simulink model "Hybrid_vehicle"  (R2020a)
settings: Solver=VariableStepAuto  StartTime=0.0  StopTime=1800  MaxStep=0.05  RelTol=1e-8
values from neighbouring files (symbols this model uses):
  Bdy_facTireFric_C = 0.018    [Model_parameters.mat]
  Bdy_lenRadiusWheel_C = 0.32    [Model_parameters.mat]
  Bdy_mEquivalentJ_C = 60    [Model_parameters.mat]
  Bdy_mVeh_C = 1400    [Model_parameters.mat]
  Bdy_vsqr2frc_C = 0.429    [Model_parameters.mat]
  Drv_facSlopeWLTC_CUR = [0 500 1000 1500 2000 2500 3000 3500 4000 4500 5000 5500 ... (98 elements, 49x2)]    [Model_parameters.mat]
  Drv_kmh2gradtqDriver_C = 200    [Model_parameters.mat]
  Drv_kmh2tqDriver_C = 500    [Model_parameters.mat]
  Drv_kmhDesWLTC_CUR = [1 2 3 4 5 6 7 8 9 10 11 12 ... (3600 elements, 1800x2)]    [Model_parameters.mat]
  Edr_pwr_LossMap_AXIS = [-150000 -100000 -60000 -35000 -23000 -7000 -2000 -1000 -200 0 200 1000 ... (19 elements, 1x19)]    [Model_parameters.mat]
  Edr_pwrInverterLosses_MAP = [19500 13000 6600 3500 2990 1470 600 450 160 50 160 450 ... (76 elements, 19x4)]    [Model_parameters.mat]
  Edr_pwrMachineLosses_MAP = [330 270 210 150 120 90 60 30 10 0 20 40 ... (209 elements, 19x11)]    [Model_parameters.mat]
  Edr_rpm_InvLossMap_AXIS = [0 2000 5000 12000]    [Model_parameters.mat]
  Edr_rpm_MachLossMap_AXIS = [0 100 200 400 1000 2000 4000 6000 8000 10000 12000]    [Model_parameters.mat]
  Edr_rpm_MaxMinTq_AXIS = [0 100 200 400 1000 2000 4000 5000 6000 7000 8000 10000 ... (13 elements, 13x1)]    [Model_parameters.mat]
  Edr_tq_MachLossMap_AXIS = [-220 -180 -140 -100 -80 -60 -40 -20 -10 0 10 20 ... (19 elements, 1x19)]    [Model_parameters.mat]
  Edr_tqEffMax_CUR = [220 220 220 220 220 220 220 180 150 125 106 81 ... (13 elements, 13x1)]    [Model_parameters.mat]
  GbxFr_tqClutchMax_C = 500    [Model_parameters.mat]
  GbxRe_facGbxReRatio_C = 10    [Model_parameters.mat]
  Ice_derfacLoadDecrease_MAP = [-5 -200 -225 -250 -275 -300 -325 -350 -375 -400 -10 -400 ... (120 elements, 10x12)]    [Model_parameters.mat]
  Ice_derfacLoadIncrease_MAP = [500 30 30 30 30 30 0 0 0 0 500 50 ... (120 elements, 10x12)]    [Model_parameters.mat]
  Ice_facEtaCocMax_MAP = [1 1 0.98 0.955 0.93 1 1 0.986 0.965 0.94 1 1 ... (35 elements, 5x7)]    [Model_parameters.mat]
  Ice_facFuelEnRich_MAP = [1 1 1 1 1 1 1 1 1 1.02 1 1 ... (35 elements, 5x7)]    [Model_parameters.mat]
  Ice_Load2TqOptIgnLamOne_MAP = [0 35 70 105 140 0 38 76 114 152 0 40 ... (35 elements, 5x7)]    [Model_parameters.mat]
  Ice_relLoad_AXIS = [0 40 80 120 160]    [Model_parameters.mat]
  Ice_relLoad_LoadDyn_AXIS = [0 80 90 100 110 120 130 140 150 160]    [Model_parameters.mat]
  Ice_relLoad_Max_CUR = [50 130 137 143 148 153 159 160 160 157 130 90]    [Model_parameters.mat]
  Ice_rpm_AXIS = [0 1000 2000 3000 4000 5000 6000]    [Model_parameters.mat]
  Ice_rpm_LoadDyn_AXIS = [500 1000 1100 1200 1300 1400 1600 2400 3000 4000 5000 6000]    [Model_parameters.mat]
  Ice_tq_AXIS = [0 40 80 120 160]    [Model_parameters.mat]
  Ice_tqLossesIce_MAP = [15 13 11 11 11 15 13 11 11 11 16 14 ... (35 elements, 5x7)]    [Model_parameters.mat]
  Ice_TqOptIgnLamOne2Load_MAP = [0 45.7 91.4 137.14 182.85 0 42.1 84.2 126.3 168.4 0 40 ... (35 elements, 5x7)]    [Model_parameters.mat]
  Pnt_capBat_C = 54000    [Model_parameters.mat]
  Pnt_facSocInit_C = 0.6    [Model_parameters.mat]
  Pnt_resBatInner_C = 0.2    [Model_parameters.mat]
libraries: simulink x2
(part 2 of 2)

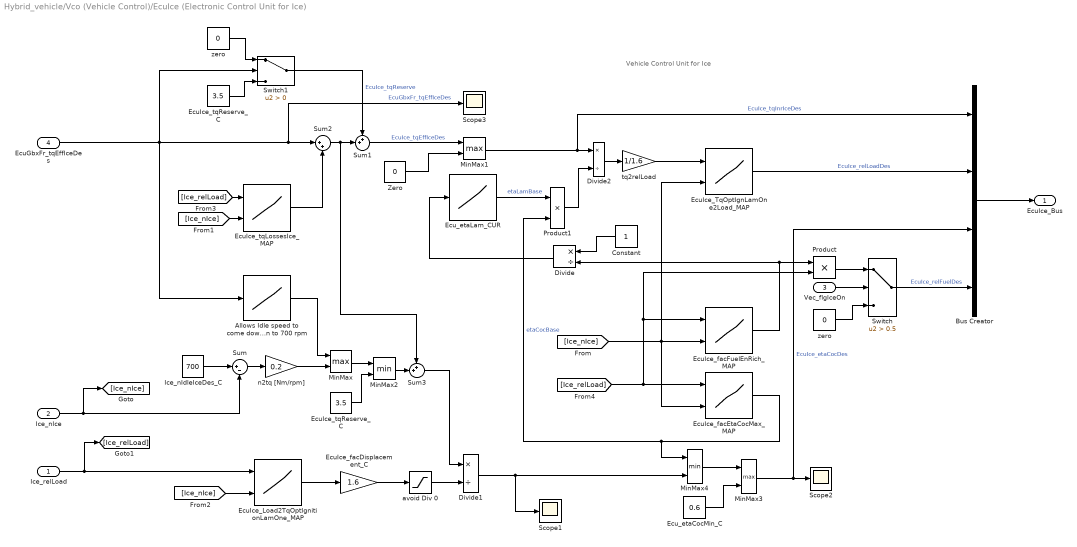
== system Hybrid_vehicle/Vco (Vehicle Control)/EcuIce (Electronic Control Unit for Ice) ==
  note: Vehicle Control Unit for Ice
  Ice_relLoad : Inport
  Ice_nIce : Inport  Port=2
  Vec_flgIceOn : Inport  Port=3
  EcuGbxFr_tqEffIceDes : Inport  Port=4
  " zero " : Constant  Value=0
  Allows Idle speed to come down to 700 rpm : Lookup_n-D  NumberOfTableDimensions=1  BreakpointsForDimension1="[-1 0  1  2]"  Table=[-1 -1 0 0 ]  InternalRulePriority=Speed  RndMeth=Simplest  InputSameDT=on
  Bus Creator : BusCreator  Inputs=4
  Constant : Constant
  Divide : Product  Inputs=*/
  Divide1 : Product  Inputs=*/
  Divide2 : Product  Inputs=*/
  EcuIce_Load2TqOptIgnitionLamOne_MAP : Lookup_n-D  BreakpointsForDimension1=Ice_relLoad_AXIS  BreakpointsForDimension2=Ice_rpm_AXIS  Table=Ice_Load2TqOptIgnLamOne_MAP  ExtrapMethod=Clip  InternalRulePriority=Speed  RndMeth=Simplest  InputSameDT=on
  EcuIce_TqOptIgnLamOne2Load_MAP : Lookup_n-D  BreakpointsForDimension1=Ice_tq_AXIS  BreakpointsForDimension2=Ice_rpm_AXIS  Table=Ice_TqOptIgnLamOne2Load_MAP  ExtrapMethod=Clip  InternalRulePriority=Speed  RndMeth=Simplest  InputSameDT=on
  EcuIce_facDisplacement_C : Gain  Gain=1.6
  EcuIce_facEtaCocMax_MAP : Lookup_n-D  BreakpointsForDimension1=Ice_relLoad_AXIS  BreakpointsForDimension2=Ice_rpm_AXIS  Table=Ice_facEtaCocMax_MAP  ExtrapMethod=Clip  InternalRulePriority=Speed  RndMeth=Simplest  InputSameDT=on
  EcuIce_facFuelEnRich_MAP : Lookup_n-D  BreakpointsForDimension1=Ice_relLoad_AXIS  BreakpointsForDimension2=Ice_rpm_AXIS  Table=Ice_facFuelEnRich_MAP  ExtrapMethod=Clip  InternalRulePriority=Speed  RndMeth=Simplest  InputSameDT=on
  EcuIce_tqLossesIce_MAP : Lookup_n-D  BreakpointsForDimension1=Ice_relLoad_AXIS  BreakpointsForDimension2=Ice_rpm_AXIS  Table=Ice_tqLossesIce_MAP  ExtrapMethod=Clip  InternalRulePriority=Speed  RndMeth=Simplest  InputSameDT=on
  EcuIce_tqReserve_C : Constant  Value=3.5
  "EcuIce_tqReserve_C " : Constant  Value=3.5
  Ecu_etaCocMin_C : Constant  Value=0.6
  Ecu_etaLam_CUR : Lookup_n-D  NumberOfTableDimensions=1  BreakpointsForDimension1="[0.5    0.6     0.7   0.8   0.85   0.9   1.0   1.1    1.2    1.3    1.4    1.5    1.6    1.7    1.8    1.9    2.0]"  Table="[0       0.5       1     1.1  1.12  1.06   1.0  0.93  0.85   0.78   0.72    0.66    0.625   0.588  0.3  0.2  0]"  ExtrapMethod=Clip  InternalRulePriority=Speed  RndMeth=Simplest  InputSameDT=on
  Ice_nIdleIceDes_C : Constant  Value=700
  MinMax : MinMax  Function=max  Inputs=2
  MinMax1 : MinMax  Function=max  Inputs=2
  MinMax2 : MinMax  Inputs=2
  MinMax3 : MinMax  Function=max  Inputs=2
  MinMax4 : MinMax  Inputs=2
  Product : Product
  Product1 : Product
  Scope1 : Scope
  Scope2 : Scope
  Scope3 : Scope
  Sum : Sum  Inputs=|+-
  Sum1 : Sum  Inputs=++|
  Sum2 : Sum  Inputs=|++
  Sum3 : Sum  Inputs=++|
  Switch : Switch  Criteria=u2 > Threshold  Threshold=0.5
  Switch1 : Switch  Criteria=u2 > Threshold
  "Zero " : Constant  Value=0
  avoid Div 0 : Saturate  UpperLimit=inf  LowerLimit=0.01
  n2tq [Nm/rpm] : Gain  Gain=0.2
  tq2relLoad : Gain  Gain=1/1.6
  "zero " : Constant  Value=0
  EcuIce_Bus : Outport  VectorParamsAs1DForOutWhenUnconnected=off
  wires:
  Bus Creator/1 -> EcuIce_Bus/1
  EcuGbxFr_tqEffIceDes/1 -> Switch1/2, Scope3/1, Sum2/1, Allows Idle speed to come down to 700 rpm/1  "EcuGbxFr_tqEffIceDes"
  Ice_nIdleIceDes_C/1 -> Sum/1
  Sum1/1 -> MinMax1/1  "EcuIce_tqEffIceDes"
  Sum3/1 -> Divide1/1
  Sum/1 -> n2tq [Nm/rpm]/1
  n2tq [Nm/rpm]/1 -> MinMax/2
  Ice_nIce/1 -> [Ice_nIce], Sum/2
  Ice_relLoad/1 -> EcuIce_Load2TqOptIgnitionLamOne_MAP/1, [Ice_relLoad]
  EcuIce_TqOptIgnLamOne2Load_MAP/1 -> Bus Creator/2  "EcuIce_relLoadDes"
  EcuIce_tqLossesIce_MAP/1 -> Sum2/2
  MinMax1/1 -> Bus Creator/1, Divide2/1  "EcuIce_tqInrIceDes"
  "Zero "/1 -> MinMax1/2
  Allows Idle speed to come down to 700 rpm/1 -> MinMax/1
  Vec_flgIceOn/1 -> Switch/2
  EcuIce_facDisplacement_C/1 -> avoid Div 0/1
  EcuIce_Load2TqOptIgnitionLamOne_MAP/1 -> EcuIce_facDisplacement_C/1
  avoid Div 0/1 -> Divide1/2
  "zero "/1 -> Switch1/1
  EcuIce_tqReserve_C/1 -> Switch1/3
  Switch1/1 -> Sum1/1  "EcuIce_tqReserve"
  Sum2/1 -> Sum3/1, Sum1/2
  Divide1/1 -> Scope1/1, MinMax4/2
  MinMax4/1 -> MinMax3/1
  Ecu_etaCocMin_C/1 -> MinMax3/2
  MinMax3/1 -> Scope2/1, Bus Creator/3  "EcuIce_etaCocDes"
  tq2relLoad/1 -> EcuIce_TqOptIgnLamOne2Load_MAP/1
  [Ice_nIce] -> EcuIce_TqOptIgnLamOne2Load_MAP/2, EcuIce_facEtaCocMax_MAP/2, EcuIce_facFuelEnRich_MAP/2
  [Ice_nIce] -> EcuIce_tqLossesIce_MAP/2
  [Ice_nIce] -> EcuIce_Load2TqOptIgnitionLamOne_MAP/2
  [Ice_relLoad] -> EcuIce_tqLossesIce_MAP/1
  MinMax/1 -> MinMax2/1
  MinMax2/1 -> Sum3/2
  "EcuIce_tqReserve_C "/1 -> MinMax2/2
  Switch/1 -> Bus Creator/4  "EcuIce_relFuelDes"
  EcuIce_facEtaCocMax_MAP/1 -> Product1/2, MinMax4/1  "etaCocBase"
  [Ice_relLoad] -> Product/2, EcuIce_facFuelEnRich_MAP/1, EcuIce_facEtaCocMax_MAP/1
  Divide2/1 -> tq2relLoad/1
  Constant/1 -> Divide/1
  Product1/1 -> Divide2/2
  Ecu_etaLam_CUR/1 -> Product1/1  "etaLamBase"
  Divide/1 -> Ecu_etaLam_CUR/1
  EcuIce_facFuelEnRich_MAP/1 -> Product/1, Divide/2
  Product/1 -> Switch/1
  " zero "/1 -> Switch/3

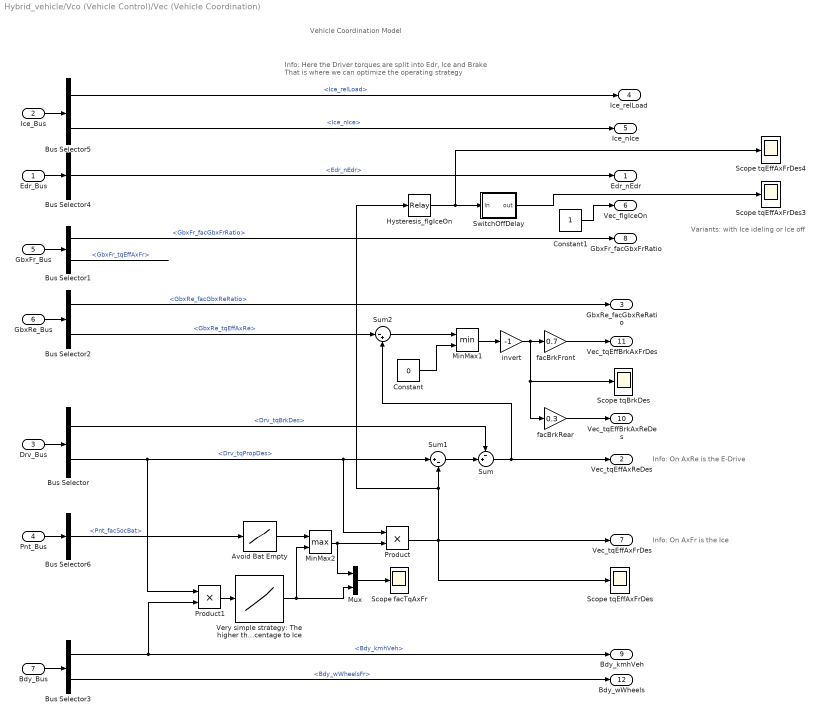
== system Hybrid_vehicle/Vco (Vehicle Control)/Vec (Vehicle Coordination) ==
  note: Vehicle Coordination Model
  note: Info: Here the Driver torques are split into Edr, Ice and Brake
      | That is where we can optimize the operating strategy
  note: Info: On AxRe is the E-Drive
  note: Info: On AxFr is the Ice
  note: Variants: with Ice ideling or Ice off
  Edr_Bus : Inport
  Ice_Bus : Inport  Port=2
  Drv_Bus : Inport  Port=3
  Pnt_Bus : Inport  Port=4
  GbxFr_Bus : Inport  Port=5
  GbxRe_Bus : Inport  Port=6
  Bdy_Bus : Inport  Port=7
  Avoid Bat Empty : Lookup_n-D  NumberOfTableDimensions=1  BreakpointsForDimension1="[0 0.1 0.2  1]"  Table="[1.1 0.8  0 0]"  InternalRulePriority=Speed  RndMeth=Simplest  InputSameDT=on
  Bus Selector : BusSelector  OutputSignals=Drv_tqBrkDes,Drv_tqPropDes
  Bus Selector1 : BusSelector  OutputSignals=GbxFr_facGbxFrRatio,GbxFr_tqEffAxFr
  Bus Selector2 : BusSelector  OutputSignals=GbxRe_facGbxReRatio,GbxRe_tqEffAxRe
  Bus Selector3 : BusSelector  OutputSignals=Bdy_kmhVeh,Bdy_wWheelsFr
  Bus Selector4 : BusSelector  OutputSignals=Edr_nEdr
  Bus Selector5 : BusSelector  OutputSignals=Ice_relLoad,Ice_nIce
  Bus Selector6 : BusSelector  OutputSignals=Pnt_facSocBat
  Constant : Constant  Value=0
  Constant1 : Constant
  Hysteresis_flgIceOn : Relay  OnSwitchValue=50  OffSwitchValue=2
  MinMax1 : MinMax  Inputs=2  ZeroCross=off
  MinMax2 : MinMax  Function=max  Inputs=2  ZeroCross=off
  Mux : Mux  Inputs=2
  Product : Product
  Product1 : Product
  Scope facTqAxFr : Scope
  Scope tqBrkDes : Scope
  Scope tqEffAxFrDes : Scope
  Scope tqEffAxFrDes3 : Scope
  Scope tqEffAxFrDes4 : Scope
  Sum : Sum  Inputs=-+|
  Sum1 : Sum  Inputs=|+-
  Sum2 : Sum  Inputs=|-+
  SwitchOffDelay : Subsystem
  "Very simple strategy: The higher the power, the more percentage to Ice" : Lookup_n-D  NumberOfTableDimensions=1  BreakpointsForDimension1="[0 2000  8000  15000  50000 200000]"  Table="[0 0  0.5 0.7  1 1]"  InternalRulePriority=Speed  RndMeth=Simplest  InputSameDT=on
  facBrkFront : Gain  Gain=0.7
  facBrkRear : Gain  Gain=0.3
  invert : Gain  Gain=-1
  Edr_nEdr : Outport  VectorParamsAs1DForOutWhenUnconnected=off
  Vec_tqEffAxReDes : Outport  Port=2  VectorParamsAs1DForOutWhenUnconnected=off
  GbxRe_facGbxReRatio : Outport  Port=3  VectorParamsAs1DForOutWhenUnconnected=off
  Ice_relLoad : Outport  Port=4  VectorParamsAs1DForOutWhenUnconnected=off
  Ice_nIce : Outport  Port=5  VectorParamsAs1DForOutWhenUnconnected=off
  Vec_flgIceOn : Outport  Port=6  VectorParamsAs1DForOutWhenUnconnected=off
  Vec_tqEffAxFrDes : Outport  Port=7  VectorParamsAs1DForOutWhenUnconnected=off
  GbxFr_facGbxFrRatio : Outport  Port=8  VectorParamsAs1DForOutWhenUnconnected=off
  Bdy_kmhVeh : Outport  Port=9  VectorParamsAs1DForOutWhenUnconnected=off
  Vec_tqEffBrkAxReDes : Outport  Port=10  VectorParamsAs1DForOutWhenUnconnected=off
  Vec_tqEffBrkAxFrDes : Outport  Port=11  VectorParamsAs1DForOutWhenUnconnected=off
  Bdy_wWheels : Outport  Port=12  VectorParamsAs1DForOutWhenUnconnected=off
  wires:
  Drv_Bus/1 -> Bus Selector/1
  Bus Selector/2 -> Sum1/1, Product/1, Product1/1  "<Drv_tqPropDes>"
  Bus Selector/1 -> Sum/1  "<Drv_tqBrkDes>"
  Sum/1 -> Vec_tqEffAxReDes/1, Sum2/2
  GbxFr_Bus/1 -> Bus Selector1/1
  Bus Selector1/1 -> GbxFr_facGbxFrRatio/1  "<GbxFr_facGbxFrRatio>"
  GbxRe_Bus/1 -> Bus Selector2/1
  Bus Selector2/1 -> GbxRe_facGbxReRatio/1  "<GbxRe_facGbxReRatio>"
  Bdy_Bus/1 -> Bus Selector3/1
  Bus Selector3/1 -> Bdy_kmhVeh/1, Product1/2  "<Bdy_kmhVeh>"
  Bus Selector3/2 -> Bdy_wWheels/1  "<Bdy_wWheelsFr>"
  Product/1 -> Vec_tqEffAxFrDes/1, Scope tqEffAxFrDes/1, Hysteresis_flgIceOn/1, Sum1/2
  Edr_Bus/1 -> Bus Selector4/1
  Bus Selector4/1 -> Edr_nEdr/1  "<Edr_nEdr>"
  Sum2/1 -> MinMax1/1
  MinMax1/1 -> invert/1
  Ice_Bus/1 -> Bus Selector5/1
  facBrkFront/1 -> Vec_tqEffBrkAxFrDes/1
  invert/1 -> Scope tqBrkDes/1, facBrkRear/1, facBrkFront/1
  facBrkRear/1 -> Vec_tqEffBrkAxReDes/1
  Constant/1 -> MinMax1/2
  Sum1/1 -> Sum/2
  Bus Selector1/2 -> ?  "<GbxFr_tqEffAxFr>"
  Bus Selector2/2 -> Sum2/1  "<GbxRe_tqEffAxRe>"
  Bus Selector5/1 -> Ice_relLoad/1  "<Ice_relLoad>"
  Bus Selector5/2 -> Ice_nIce/1  "<Ice_nIce>"
  Hysteresis_flgIceOn/1 -> Scope tqEffAxFrDes4/1, SwitchOffDelay/1(In)
  SwitchOffDelay/1(out) -> Scope tqEffAxFrDes3/1
  Product1/1 -> "Very simple strategy: The higher the power, the more percentage to Ice"/1
  Constant1/1 -> Vec_flgIceOn/1
  Pnt_Bus/1 -> Bus Selector6/1
  Bus Selector6/1 -> Avoid Bat Empty/1  "<Pnt_facSocBat>"
  MinMax2/1 -> Mux/1, Product/2
  "Very simple strategy: The higher the power, the more percentage to Ice"/1 -> MinMax2/2, Mux/2
  Mux/1 -> Scope facTqAxFr/1
  Avoid Bat Empty/1 -> MinMax2/1

== system Hybrid_vehicle/Vco (Vehicle Control)/Vec (Vehicle Coordination)/SwitchOffDelay ==
  In : Inport
  Constant1 : Constant
  Integrator : Integrator  ExternalReset=level
  Relational Operator : RelationalOperator  Operator=<  OutDataTypeStr=boolean  RndMeth=Simplest
  TimeDelay : Constant  Value=4
  out : Outport  VectorParamsAs1DForOutWhenUnconnected=off
  wires:
  Relational Operator/1 -> out/1
  Constant1/1 -> Integrator/1
  In/1 -> Integrator/2
  Integrator/1 -> Relational Operator/1
  TimeDelay/1 -> Relational Operator/2
